simulink subsystem "Filter"  (R2019b)
settings: Solver=VariableStepAuto  StartTime=0.0  StopTime=10.0  RelTol=1e-3
model mask{num=[1 0], den=[1 0]}
  mask prompts: num "Numerator"; den "Denominator"
undefined symbols (not defined in the file): dt_control
settings Model: Creator=giaco  LastModifiedBy=giaco

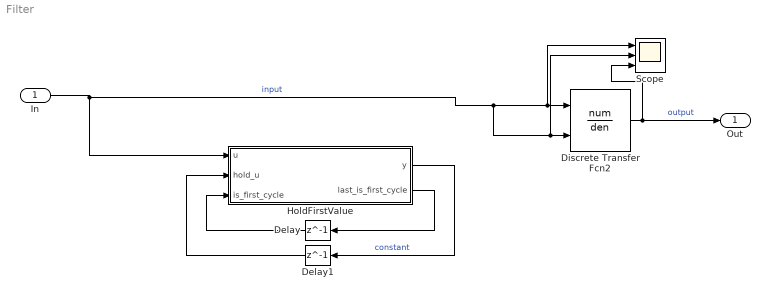
== system Filter ==
  In : Inport
  Delay : Delay  DelayLength=1  InitialCondition=1
  Delay1 : Delay  DelayLength=1  InitialCondition=1
  Discrete Transfer Fcn2 : DiscreteTransferFcn  Numerator=num  Denominator=den  InitialStatesSource=Input port  SampleTime=dt_control
      settings: InputPortMap=u0,p5
  HoldFirstValue : MATLAB Function  TreatAsAtomicUnit=on
  Scope : Scope  NumInputPorts=3
  Out : Outport
  wires:
  Discrete Transfer Fcn2/1 -> Out/1, Scope/3  "output"
  HoldFirstValue/1(y) -> Delay1/1  "constant"
  In/1 -> HoldFirstValue/1(u), Discrete Transfer Fcn2/1, Scope/1, Discrete Transfer Fcn2/2, Scope/2  "input"
  Delay/1 -> HoldFirstValue/3(is_first_cycle)
  HoldFirstValue/2(last_is_first_cycle) -> Delay/1
  Delay1/1 -> HoldFirstValue/2(hold_u)

== matlab function Filter/HoldFirstValue ==
  data: u input; y output; hold_u input; is_first_cycle input; last_is_first_cycle output
function [y,last_is_first_cycle]  = holdFirstValue(u, hold_u, is_first_cycle)

if is_first_cycle
    y = u;
else
    y = hold_u;
end
last_is_first_cycle = 0;

end
